simulink model "model"  (R2014a)
settings: Solver=ode45  StartTime=0.0  StopTime=10.0  RelTol=1e-3
values from neighbouring files (symbols this model uses):
  g0 = 9.81    [Calculations.m]
  mu = 3.5316*10^12    (= 3531600000000)    [Calculations.m]
  R = 600000    [Calculations.m]
  R_vac = 670000    [Calculations.m]
  s0 = [R,0,0]    [Calculations.m]
  v0 = [0,0,0]    [Calculations.m]
  w_rot = -174.9425/600000    (= -0.000291570833333)    [Calculations.m]
undefined symbols (not defined in the file or in its folder): magnitude
libraries: aerolibtransform2 x1
settings Model: Creator=Frederic  LastModifiedBy=Frederic
settings SolverCC: MaxConsecutiveMinStep=1000
settings DataIOCC: LimitDataPoints=off  SaveFormat=Structure  TimeSaveName=t  OutputSaveName=out

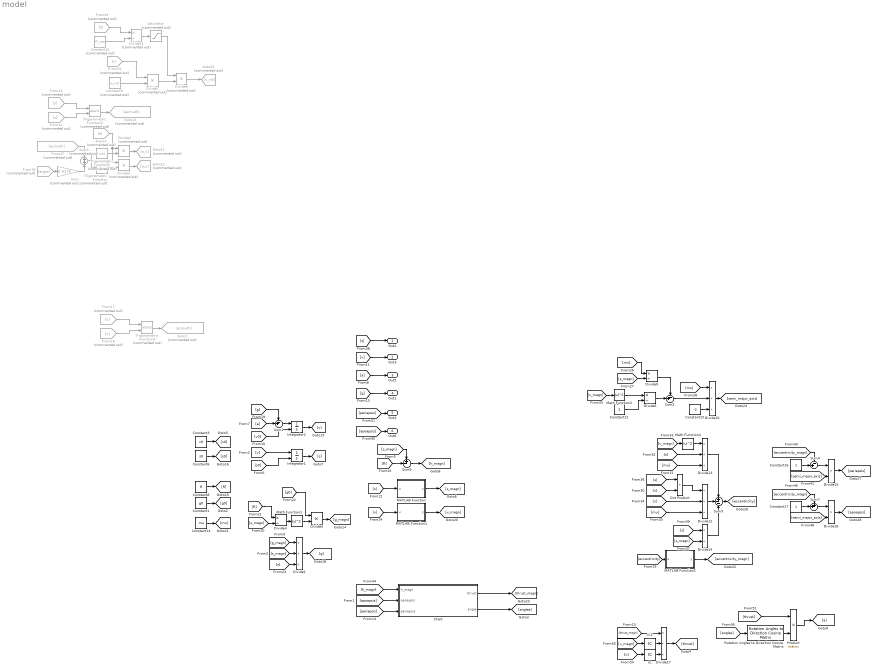
== system model ==
  Chart : Stateflow chart  TreatAsAtomicUnit=on
  Constant1 : Constant  Value=g0
  Constant10 : Constant  Commented=on  Value=R_vac
  Constant12 : Constant  Value=2
  Constant14 : Constant  Value=mu
  Constant15 : Constant  Value=-2
  Constant16 : Constant
  Constant17 : Constant
  Constant3 : Constant  Value=v0  VectorParams1D=off
  Constant6 : Constant  Value=s0  VectorParams1D=off
  Constant8 : Constant  Value=R  VectorParams1D=off
  Constant9 : Constant  Commented=on  Value=w_rot
  Divide1 : Product  Inputs=*/*
  Divide10 : Product  Inputs=*//
  Divide11 : Product  Commented=on  Inputs=*/
  Divide12 : Product  Inputs=**/
  Divide13 : Product  Inputs=**/
  Divide{4,6,9,14} (4 alike) : Product  Inputs=*/
  Divide15 : Product  Inputs=**
  Divide16 : Product  Inputs=**
  Divide17 : Product  Inputs=*/*
  Divide{2..3,7..8} (4 alike) : Product  Commented=on  Inputs=**
  Divide5 : Product  Inputs=**
  Dot Product : DotProduct  InputSameDT=on  OutDataTypeStr=Inherit: Inherit via internal rule
  From16 : From  Commented=on  GotoTag=x
  From17 : From  Commented=on  GotoTag=y
  From18 : From  Commented=on  GotoTag=angle
  From4 : From  Commented=on  GotoTag=a
  From42 : From  Commented=on  GotoTag=x
  From43 : From  Commented=on  GotoTag=y
  From47 : From  Commented=on  GotoTag=azimuth
  From49 : From  Commented=on  GotoTag=h
  From53 : From  Commented=on  GotoTag=r
  Gain : Gain  Commented=on  Gain=0.0175
  Goto1 : Goto  Commented=on  GotoTag=azimuth
  Goto11 : Goto  Commented=on  GotoTag=a_x
  Goto12 : Goto  Commented=on  GotoTag=a_y
  Goto13 : Goto  Commented=on  GotoTag=azimuth
  Goto25 : Goto  Commented=on  GotoTag=v_rot
  IC : InitialCondition  Value=[1 0 0]
  IC1 : InitialCondition
  Integrator1 : Integrator  InitialConditionSource=external
  Integrator2 : Integrator  InitialConditionSource=external
  MATLAB Function : MATLAB Function  TreatAsAtomicUnit=on
  MATLAB Function1 : MATLAB Function  TreatAsAtomicUnit=on
  MATLAB Function2 : MATLAB Function  TreatAsAtomicUnit=on
  Math Function1 : Math  Operator=magnitude^2  SaturateOnIntegerOverflow=on
  Math Function2 : Math  Operator=magnitude^2  SaturateOnIntegerOverflow=on
  Math Function4 : Math  Operator=magnitude^2  SaturateOnIntegerOverflow=on
  Product : Product  Multiplication=Matrix(*)
  Rotation Angles to Direction Cosine Matrix : aerolibtransform2/Rotation Angles to Direction Cosine Matrix  rotationOrder=ZXY
  Saturation : Saturate  Commented=on  UpperLimit=1  LowerLimit=0
  Sum1 : Sum  Inputs=-+|
  Sum2 : Sum  Inputs=-+|
  Sum3 : Sum  Inputs=+--
  Sum4 : Sum  Inputs=-+|
  Sum5 : Sum  Commented=on  Inputs=+|+
  Sum6 : Sum  Inputs=+-|
  Sum7 : Sum  Inputs=++|
  Trigonometric Function : Trigonometry  Commented=on
  Trigonometric Function1 : Trigonometry  Commented=on  Operator=cos
  Trigonometric Function2 : Trigonometry  Commented=on  Operator=atan2
  Trigonometric Function3 : Trigonometry  Commented=on  Operator=atan2
  Out2 : Outport
  Out3 : Outport  Port=2
  Out5 : Outport  Port=3
  Out1 : Outport  Port=4
  Out4 : Outport  Port=5
  Out6 : Outport  Port=6
  wires:
  Constant1/1 -> [g0]
  [s] -> Out2/1
  [v] -> Out3/1
  From4/1 -> Divide2/1, Divide3/1
  [a] -> Out5/1
  Trigonometric Function1/1 -> Divide2/2
  Trigonometric Function/1 -> Divide3/2
  Divide2/1 -> Goto11/1
  Divide3/1 -> Goto12/1
  Constant8/1 -> [R]
  From18/1 -> Gain/1
  Sum5/1 -> Trigonometric Function/1, Trigonometric Function1/1
  Gain/1 -> Sum5/2
  From47/1 -> Sum5/1
  [h_magn] -> Chart/1(h_magn)
  Chart/1(thrust) -> [thrust_magn]
  Chart/2(angle) -> [angles]
  [s_magn] -> Sum6/1
  [R] -> Sum6/2
  Sum6/1 -> [h_magn]
  From42/1 -> Trigonometric Function2/2
  From43/1 -> Trigonometric Function2/1
  Trigonometric Function2/1 -> Goto13/1
  Constant9/1 -> Divide7/2
  From53/1 -> Divide7/1
  Divide7/1 -> Divide8/2
  Divide8/1 -> Goto25/1
  From49/1 -> Divide11/1
  Divide11/1 -> Saturation/1
  Constant10/1 -> Divide11/2
  Saturation/1 -> Divide8/1
  Constant3/1 -> [v0]
  Constant6/1 -> [s0]
  [s] -> MATLAB Function/1(u)
  MATLAB Function/1(y) -> [s_magn]
  [g] -> Out1/1
  [v] -> Integrator1/1
  [s0] -> Integrator1/2
  [v0] -> Integrator2/2
  [a] -> Sum1/2
  Sum1/1 -> Integrator2/1
  [g] -> Sum1/1
  [g0] -> Divide5/1
  Math Function1/1 -> Divide5/2
  Divide4/1 -> Math Function1/1
  [R] -> Divide4/1
  Integrator1/1 -> [s]
  Integrator2/1 -> [v]
  [s_magn] -> Divide4/2
  Divide5/1 -> [g_magn]
  [g_magn] -> Divide1/1
  [s_magn] -> Divide1/2
  [s] -> Divide1/3
  Divide1/1 -> [g]
  [v] -> MATLAB Function1/1(u)
  MATLAB Function1/1(y) -> [v_magn]
  [v_magn] -> Math Function2/1
  Math Function2/1 -> Divide6/1
  Constant12/1 -> Divide6/2
  Divide6/1 -> Sum2/2
  Constant14/1 -> [mu]
  [mu] -> Divide9/1
  [s_magn] -> Divide9/2
  Divide9/1 -> Sum2/1
  [mu] -> Divide10/1
  Sum2/1 -> Divide10/2
  Divide10/1 -> [semi_major_axis]
  Constant15/1 -> Divide10/3
  [v] -> Dot Product/2
  Divide12/1 -> Sum3/2
  Math Function4/1 -> Divide13/1
  [s] -> Divide13/2
  Divide13/1 -> Sum3/1
  Sum3/1 -> [eccentricity]
  [v_magn] -> Math Function4/1
  [mu] -> Divide13/3
  [s] -> Dot Product/1
  Dot Product/1 -> Divide12/1
  [v] -> Divide12/2
  [mu] -> Divide12/3
  [s] -> Divide14/1
  [s_magn] -> Divide14/2
  Divide14/1 -> Sum3/3
  [eccentricity] -> MATLAB Function2/1(u)
  MATLAB Function2/1(y) -> [eccentricity_magn]
  Constant16/1 -> Sum4/2
  [eccentricity_magn] -> Sum4/1
  Sum4/1 -> Divide15/1
  [semi_major_axis] -> Divide15/2
  Divide15/1 -> [periapsis]
  Constant17/1 -> Sum7/2
  [eccentricity_magn] -> Sum7/1
  Sum7/1 -> Divide16/1
  [semi_major_axis] -> Divide16/2
  Divide16/1 -> [apoapsis]
  [periapsis] -> Out4/1
  [apoapsis] -> Out6/1
  [apoapsis] -> Chart/2(apoapsis)
  [periapsis] -> Chart/3(periapsis)
  From16/1 -> Trigonometric Function3/2
  From17/1 -> Trigonometric Function3/1
  Trigonometric Function3/1 -> Goto1/1
  [thrust_magn] -> Divide17/1
  Divide17/1 -> [thrust]
  IC1/1 -> Divide17/2
  [v_magn] -> IC1/1
  [v] -> IC/1
  IC/1 -> Divide17/3
  Product/1 -> [a]
  Rotation Angles to Direction Cosine Matrix/1 -> Product/2
  [angles] -> Rotation Angles to Direction Cosine Matrix/1
  [thrust] -> Product/1

== matlab function model/MATLAB Function1 ==
  data: u input; y output
function y = magn(u)
y = sqrt(sum(abs(u).^2,2));

== matlab function model/MATLAB Function ==
  data: u input; y output
function y = magn(u)
y = sqrt(sum(abs(u).^2,2));

== stateflow chart model/Chart ==
  state state001
    entry:
    thrust = 20;
    angle = [0,0,0]*0.0175;
  state state002
    entry:
    thrust = 20;
    angle = [20,0,0]*0.0175;
  state state003
    entry:
    thrust = 20;
    angle = [45,0,0]*0.0175;
  state state007
    entry:
    thrust = 0;
    angle = [90,0,0]*0.0175;
  state state004
    entry:
    thrust = 20;
    angle =  [90,0,0]*0.0175;
  state state005
    entry:
    thrust = 0;
    angle =  [90,0,0]*0.0175;
  state state006
    entry:
    thrust = 15;
    angle = [90,0,0]*0.0175;
  state state008
    entry:
    thrust = 0;
    angle = [90,0,0]*0.0175;
  (default) -> state001
  state001 -> state002 : [h_magn>10000]
  state002 -> state003 : [h_magn>40000]
  state007 -> state003 [order 1] : [apoapsis<=700000]
  state003 -> state007 [order 2] : [apoapsis>700000]
  state003 -> state004 [order 1] : [h_magn>70000]
  state007 -> state006 [order 2] : [h_magn>90000]
  state004 -> state005 : [apoapsis>700000 && h_magn>70000]
  state005 -> state006 : [h_magn>90000]
  state006 -> state008 : [periapsis>700000]
  data: h_magn input; thrust output; angle output; apoapsis input; periapsis input

== matlab function model/MATLAB Function2 ==
  data: u input; y output
function y = magn(u)
y = sqrt(sum(abs(u).^2,2));
